simulink model "euler2quaternion"  (Simulink 8.7)
settings: Solver=VariableStepAuto  StartTime=0.0  StopTime=10.0  RelTol=1e-3
settings Model: Creator=mgreiff  LastModifiedBy=mgreiff
settings DataIOCC: LimitDataPoints=off  SaveFormat=Dataset
settings DebuggingCC: UnderspecifiedInitializationDetection=Simplified  MergeDetectMultiDrivingBlocksExec=error
settings HardwareCC: ProdBitPerPointer=64  ProdLargestAtomicFloat=Float  ProdIntDivRoundTo=Zero  ProdEndianess=LittleEndian  ProdWordSize=64  ProdHWDeviceType=Intel->x86-64 (Windows64)
settings ModelReferenceCC: PropagateSignalLabelsOutOfModel=on
settings ConfigComp: CovModelRefEnable=off

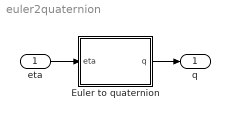
== system euler2quaternion ==
  eta : Inport  PortDimensions=3
  Euler to quaternion : MATLAB Function  TreatAsAtomicUnit=on
  q : Outport  PortDimensions=4
  wires:
  eta/1 -> Euler to quaternion/1(eta)
  Euler to quaternion/1(q) -> q/1

== matlab function Euler to quaternion ==
  data: eta input double; q output double
function q = fcn(eta)
%#codegen
phi=  eta(1);
theta = eta(2);
psi = eta(3);

cphi = cos(phi/2);
sphi = sin(phi/2);


ctheta = cos(theta/2);
stheta = sin(theta/2);

cpsi = cos(psi/2);
spsi = sin(psi/2);

q = [cphi*ctheta*cpsi + sphi*stheta*spsi;
     sphi*ctheta*cpsi - cphi*stheta*spsi;
     cphi*stheta*cpsi + sphi*ctheta*spsi;
     cphi*ctheta*spsi - sphi*stheta*cpsi];
 
if cos(phi)*cos(theta) < 0
    q = q;
end
